simulink model "pwmModule"  (R2018b)
settings: Solver=VariableStepAuto  StartTime=0.0  StopTime=0.01  RelTol=1e-3
libraries: simulink x2, powerlib_meascontrol x1
settings Model: Creator=K2  LastModifiedBy=K2

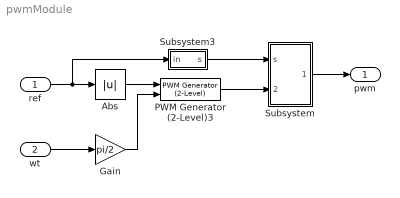
== system pwmModule ==
  ref : Inport
  wt : Inport  Port=2
  Abs : Abs
  Gain : Gain  Gain=pi/2
  PWM Generator (2-Level)3 : powerlib_meascontrol/Pulse & Signal Generators/PWM Generator (2-Level)  ModulatorType=Single-phase half-bridge (2 pulses)  ModulatorMode=Synchronized  Fc=freq  Pc=0  nF=1  MinMax=[0 1]  SamplingTechnique=Natural  ModulatingSignals=off  m=0.8  Freq=60  Phase=0  Ts=-1  ShowCarrierOutport=off
      settings: SourceProductName=Simscape Power Systems
  Subsystem : Subsystem
  Subsystem3 : Subsystem
  pwm : Outport
  wires:
  PWM Generator (2-Level)3/1 -> Subsystem/2(pwm in)
  ref/1 -> Abs/1, Subsystem3/1(in)
  Subsystem3/1(s) -> Subsystem/1(s)
  Subsystem/1(pwm) -> pwm/1
  Abs/1 -> PWM Generator (2-Level)3/1
  wt/1 -> Gain/1
  Gain/1 -> PWM Generator (2-Level)3/2

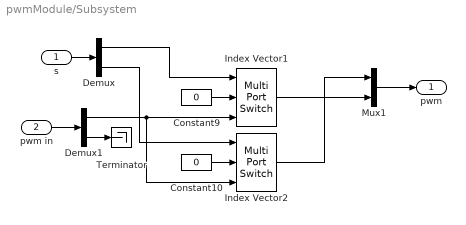
== system pwmModule/Subsystem ==
  s : Inport
  pwm in : Inport  Port=2
  Constant10 : Constant  Value=0
  Constant9 : Constant  Value=0
  Demux : Demux  Outputs=2
  Demux1 : Demux  Outputs=2
  Index Vector1 : MultiPortSwitch  DataPortOrder=Zero-based contiguous  Inputs=2  zeroidx=on
  Index Vector2 : MultiPortSwitch  DataPortOrder=Zero-based contiguous  Inputs=2  zeroidx=on
  Mux1 : Mux  Inputs=2
  Terminator : Terminator
  pwm : Outport
  wires:
  Demux1/1 -> Index Vector2/3, Index Vector1/3
  Index Vector2/1 -> Mux1/1
  Index Vector1/1 -> Mux1/2
  Demux/1 -> Index Vector1/1
  Demux/2 -> Index Vector2/1
  pwm in/1 -> Demux1/1
  Constant9/1 -> Index Vector1/2
  Constant10/1 -> Index Vector2/2
  Demux1/2 -> Terminator/1
  Mux1/1 -> pwm/1
  s/1 -> Demux/1

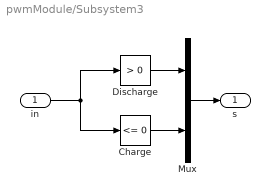
== system pwmModule/Subsystem3 ==
  in : Inport
  Charge : simulink/Logic and Bit Operations/Compare To Constant  relop=<=  const=0  OutDataTypeStr=boolean
  Discharge : simulink/Logic and Bit Operations/Compare To Constant  relop=>  const=0  OutDataTypeStr=boolean
  Mux : Mux  Inputs=2
  s : Outport
  wires:
  in/1 -> Charge/1, Discharge/1
  Charge/1 -> Mux/2
  Discharge/1 -> Mux/1
  Mux/1 -> s/1
